simulink model "Test_Tricopter_Model"  (R2015a)
settings: Solver=ode3  SolverMode=SingleTasking  StartTime=0.0  StopTime=20  FixedStep=T_sim  RelTol=1e-3
PreLoadFcn:
  | LoadLibraries
values from neighbouring files (symbols this model uses):
  a = 10.26    [SetupComplete.m]
  A_x = 0.015    [SetupComplete.m]
  A_y = A_x    (= 0.015)    [SetupComplete.m]
  A_z = 0.16    [SetupComplete.m]
  C_d0 = 0.001193    [SetupComplete.m]
  C_x = 1.2    [SetupComplete.m]
  C_y = C_x    (= 1.2)    [SetupComplete.m]
  C_z = 2.2    [SetupComplete.m]
  CG_0 = [0,0,0.02]'    [SetupComplete.m]
  g = 9.81    [SetupComplete.m]
  h = 0.08    [SetupComplete.m]
  h_FA = 0.02    [SetupComplete.m]
  h_M = 0.064    [SetupComplete.m]
  I_BAC_0 = [ Ix,0,Ixz;0,Iy,0;Ixz,0,Iz]    [SetupComplete.m]
  I_prop = 1/4*M_eq*R^2*diag([1,1,2])    [SetupComplete.m]
  I_tube = [1/2*M_tube*R_tube_eq^2,0,  0  ;           0 ,1/3*M_tube*l_arm^2,0;             0  ,0,1/3*M_tube*l_arm^2]    [SetupComplete.m]
  Initial_Omegas = [1;1;1]*Omega_hover    [Run3Copter.m]
  J_FA = I_prop(1,1) + m_prop*h^2  + m_FA*h_FA^2 + m_M*h_M^2    [SetupComplete.m]
  J_T = J_m+1/2*M_eq*R^2    (= 2.000642e-05)    [SetupComplete.m]
  Ki = lqi(LM_4DOF_aug, Q,R)    [robust_controller.m]
  l = 0.3450    (= 0.345)    [NDI_components.m]    (also in SetupComplete.m; robust_controller.m)
  l_arm = 0.264    [SetupComplete.m]
  m = 3.51    [SetupComplete.m]
  m_0 = 2.61    [SetupComplete.m]
  m_FA = 0.02    [SetupComplete.m]
  m_M = 0.300    (= 0.3)    [SetupComplete.m]
  m_prop = 0.02    [SetupComplete.m]
  R = 0.1778    [SetupComplete.m]    (also in robust_controller.m = eye(4))
  rho = 1.15    [SetupComplete.m]
  sigma = b*c/(pi*R)    (= 0.107416159567)    [SetupComplete.m]
  T_sim = 0.01    [Run3Copter.m]
  theta_0 = 0.38397    [SetupComplete.m]
  theta_1 = -0.2967    [SetupComplete.m]
  trim_simplemodel = [0.589627915568 -2.20656039197 0 0.588313336084 0 0 0.588313330414 0 0]    [trimvalues.mat]
  V_4DOF_last = [0.0122475086001 0.00870447045314 -0.0292257707267 -0.0198753669721 -0.00290766514824 -0.0269511839788 0.0344308792695 -0.0305235710433 -0.0274078219028 -0.0329291952852 -0.0272335702183 -0.00643013158961 ... (1500 elements, 50x30)]    [NN_c_weights.mat]
  v_i0 = sqrt( 1/3*m*g/(2*rho*pi*R^2)  )    [SetupComplete.m]
  W_4DOF_last = [0.0132359246225 -0.0402459595001 -0.0221501781133 0.0046881519205 0.0457506835434 0.0464888535199 -0.0342386918322 0.0470592781761 0.0457166948243 -0.00146243512772 0.0300280468889 -0.0358113661373 ... (204 elements, 4x51)]    [NN_c_weights.mat]
undefined symbols (not defined in the file or in its folder): DOWN_0, EAST_0, Motor, NORTH_0, P_0, Prop, Q_0, R_0, sigmatest, U_0, V_0, v_i_adim, Vx_adim, Vz_adim, W_0
undefined symbols (not defined in the file): Initial_Torques, Rotation_sign, Tau_motors
libraries: simulink x61, XXCopter x32, vrlib x26, simulink_extras x6, aerolib6dofsys x3, qcatlib x3, dspinverses x3, lib_controller x2, aerolibtransform2 x2, aerolib6dof2 x1
(part 10 of 10)

== matlab function Test_Tricopter_Model/Controller/NDI+CA Controller/4DOF NDI+CA Controller - No massic update/G(X) 4DOF_WPQR1 ==
  data: gx output size=[4,4]; prev_input input size=[9,1]
function gx = gx(prev_input)
    % Calculates f_hat(x). The expression is calculated in NDI_components
    % x_dot = f(x) + g(x,u)
    %   g(x,u) ~= g(x,u0) + jac(g(x,u), u)(u0) * (u - u0)
    %   g(x,u) ~= h(x,u0) + jac(g(x,u), u)(u0) * u
    % x_dot = f_hat(x) + jac(g(x,u), u) * u
    %   f_hat(x) = f(x) + g(x,u0) - jac(g(x,u), u)(u0) *  u0
    %   g_hat(x) = jac(g(x,u), u)(u0)
    % x_dot = f_hat(x) + g_hat(x) * u
    tau1_0 = prev_input(1);
    eta1_0 = prev_input(2);
    gamma1_0 = prev_input(3);
    tau2_0 = prev_input(4);
    eta2_0 = prev_input(5);
    gamma2_0 = prev_input(6);
    tau3_0 = prev_input(7);
    eta3_0 = prev_input(8);
    gamma3_0 = prev_input(9);
    
    % This matrix was precomputed in NDI_components.m
    % TODO Precompute sines and cosines to improve performance. Some
    % repeated terms can also be precomputed
    
    % Kt = 29.6 Kq = 0.3
    gx = [...
                          -7.379*cos(eta1_0),                                7.379*tau1_0*sin(eta1_0), -7.379,  -7.379;
     0.04359*cos(eta1_0) - 1.541*sin(eta1_0), - 1.541*tau1_0*cos(eta1_0) - 0.04359*tau1_0*sin(eta1_0), -48.41,   48.32;
       43.76*cos(eta1_0) + 1.469*sin(eta1_0),     1.469*tau1_0*cos(eta1_0) - 43.76*tau1_0*sin(eta1_0), -21.88,  -21.88;
       26.0*sin(eta1_0) - 0.8729*cos(eta1_0),     26.0*tau1_0*cos(eta1_0) + 0.8729*tau1_0*sin(eta1_0),  1.997, -0.2515];
 
% Kt = 15 Kq = 0.07
%                        -4.274*cos(eta1_0),                                 4.274*tau1_0*sin(eta1_0), -4.274,  -4.274;
%  0.01017*cos(eta1_0) - 0.8926*sin(eta1_0), - 0.8926*tau1_0*cos(eta1_0) - 0.01017*tau1_0*sin(eta1_0), -28.02,    28.0;
%    25.34*cos(eta1_0) + 0.3428*sin(eta1_0),     0.3428*tau1_0*cos(eta1_0) - 25.34*tau1_0*sin(eta1_0), -12.67,  -12.67;
%    15.06*sin(eta1_0) - 0.2037*cos(eta1_0),     15.06*tau1_0*cos(eta1_0) + 0.2037*tau1_0*sin(eta1_0), 0.8549, -0.4475];

== matlab function Test_Tricopter_Model/Controller/NDI+CA Controller/4DOF NDI+CA Controller - No massic update/Rotational Kinematics ==
  data: PQR output; Eulerdot input; Euler input
function PQR = rot_kin(Eulerdot,Euler)
%solves rotational kinematic equations
Phi = Euler(1);
Theta = Euler(2);
Psi = Euler(3);
A = [1 sin(Phi)*tan(Theta) cos(Phi)*tan(Theta);
     0 cos(Phi) -sin(Phi);
     0 sin(Phi)*sec(Theta) cos(Phi)*sec(Theta)];
PQR = A'*Eulerdot;
end

== matlab function Test_Tricopter_Model/3 Copter Complete/Arms Dynamics: Forces and Moments/9 DOF Arms Dynamics: Forces and Moments/9 DOF Arms Dynamics: Forces and Moments/Arm Dynamics1/Gyroscopic Moments/Arm Inertia1 ==
  data: T_FAFb input; Arm_axis input; J_Arm output; I_tube parameter; I_prop parameter; h_FA parameter; h_M parameter; m_FA parameter; m_M parameter; m_prop parameter; h parameter
function J_Arm  = Arm_inertia(T_FAFb,Arm_axis, I_tube, I_prop, h_FA, h_M, m_FA, m_M, m_prop, h)


r_FAO=Arm_axis+T_FAFb*[0;0;-h_FA];
r_MO=Arm_axis+T_FAFb*[0;0;-h_M];
r_po=Arm_axis+T_FAFb*[0;0;-h];

I_FA = m_FA*[ r_FAO(2)^2+r_FAO(3)^2,r_FAO(1)*r_FAO(2),r_FAO(1)*r_FAO(3);...
            r_FAO(1)*r_FAO(2), r_FAO(1)^2+r_FAO(3)^2, r_FAO(2)*r_FAO(3);...
            r_FAO(1)*r_FAO(3),r_FAO(2)*r_FAO(3), r_FAO(1)^2+r_FAO(2)^2];
I_M = m_M*[ r_MO(2)^2+r_MO(3)^2,r_MO(1)*r_MO(2),r_MO(1)*r_MO(3);...
            r_MO(1)*r_MO(2), r_MO(1)^2+r_MO(3)^2, r_MO(2)*r_MO(3);...
            r_MO(1)*r_MO(3),r_MO(2)*r_MO(3), r_MO(1)^2+r_MO(2)^2];
I_steiner = m_prop*[ r_po(2)^2+r_po(3)^2,r_po(1)*r_po(2),r_po(1)*r_po(3);...
            r_po(1)*r_po(2), r_po(1)^2+r_po(3)^2, r_po(2)*r_po(3);...
            r_po(1)*r_po(3),r_po(2)*r_po(3), r_po(1)^2+r_po(2)^2];


% J_Arm = T_FAFb*I_prop*T_FAFb'+ I_tube +I_FA+I_M+I_steiner;
J_Arm = T_FAFb*I_prop*T_FAFb' +I_FA+I_M+I_steiner; % Quitamos el tubo ya que es insignificante y hay que calcularlo para cada brazo

== matlab function Test_Tricopter_Model/3 Copter Complete/Arms Dynamics: Forces and Moments/9 DOF Arms Dynamics: Forces and Moments/9 DOF Arms Dynamics: Forces and Moments/Arm Dynamics2/Gyroscopic Moments/Arm Inertia1 ==
  data: T_FAFb input; Arm_axis input; J_Arm output; I_tube parameter; I_prop parameter; h_FA parameter; h_M parameter; m_FA parameter; m_M parameter; m_prop parameter; h parameter
function J_Arm  = Arm_inertia(T_FAFb,Arm_axis, I_tube, I_prop, h_FA, h_M, m_FA, m_M, m_prop, h)


r_FAO=Arm_axis+T_FAFb*[0;0;-h_FA];
r_MO=Arm_axis+T_FAFb*[0;0;-h_M];
r_po=Arm_axis+T_FAFb*[0;0;-h];

I_FA = m_FA*[ r_FAO(2)^2+r_FAO(3)^2,r_FAO(1)*r_FAO(2),r_FAO(1)*r_FAO(3);...
            r_FAO(1)*r_FAO(2), r_FAO(1)^2+r_FAO(3)^2, r_FAO(2)*r_FAO(3);...
            r_FAO(1)*r_FAO(3),r_FAO(2)*r_FAO(3), r_FAO(1)^2+r_FAO(2)^2];
I_M = m_M*[ r_MO(2)^2+r_MO(3)^2,r_MO(1)*r_MO(2),r_MO(1)*r_MO(3);...
            r_MO(1)*r_MO(2), r_MO(1)^2+r_MO(3)^2, r_MO(2)*r_MO(3);...
            r_MO(1)*r_MO(3),r_MO(2)*r_MO(3), r_MO(1)^2+r_MO(2)^2];
I_steiner = m_prop*[ r_po(2)^2+r_po(3)^2,r_po(1)*r_po(2),r_po(1)*r_po(3);...
            r_po(1)*r_po(2), r_po(1)^2+r_po(3)^2, r_po(2)*r_po(3);...
            r_po(1)*r_po(3),r_po(2)*r_po(3), r_po(1)^2+r_po(2)^2];


% J_Arm = T_FAFb*I_prop*T_FAFb'+ I_tube +I_FA+I_M+I_steiner;
J_Arm = T_FAFb*I_prop*T_FAFb' +I_FA+I_M+I_steiner; % Quitamos el tubo ya que es insignificante y hay que calcularlo para cada brazo

== matlab function Test_Tricopter_Model/3 Copter Complete/Arms Dynamics: Forces and Moments/9 DOF Arms Dynamics: Forces and Moments/9 DOF Arms Dynamics: Forces and Moments/Arm Dynamics/Gyroscopic Moments/Arm Inertia1 ==
  data: T_FAFb input; Arm_axis input; J_Arm output; I_tube parameter; I_prop parameter; h_FA parameter; h_M parameter; m_FA parameter; m_M parameter; m_prop parameter; h parameter
function J_Arm  = Arm_inertia(T_FAFb,Arm_axis, I_tube, I_prop, h_FA, h_M, m_FA, m_M, m_prop, h)


r_FAO=Arm_axis+T_FAFb*[0;0;-h_FA];
r_MO=Arm_axis+T_FAFb*[0;0;-h_M];
r_po=Arm_axis+T_FAFb*[0;0;-h];

I_FA = m_FA*[ r_FAO(2)^2+r_FAO(3)^2,r_FAO(1)*r_FAO(2),r_FAO(1)*r_FAO(3);...
            r_FAO(1)*r_FAO(2), r_FAO(1)^2+r_FAO(3)^2, r_FAO(2)*r_FAO(3);...
            r_FAO(1)*r_FAO(3),r_FAO(2)*r_FAO(3), r_FAO(1)^2+r_FAO(2)^2];
I_M = m_M*[ r_MO(2)^2+r_MO(3)^2,r_MO(1)*r_MO(2),r_MO(1)*r_MO(3);...
            r_MO(1)*r_MO(2), r_MO(1)^2+r_MO(3)^2, r_MO(2)*r_MO(3);...
            r_MO(1)*r_MO(3),r_MO(2)*r_MO(3), r_MO(1)^2+r_MO(2)^2];
I_steiner = m_prop*[ r_po(2)^2+r_po(3)^2,r_po(1)*r_po(2),r_po(1)*r_po(3);...
            r_po(1)*r_po(2), r_po(1)^2+r_po(3)^2, r_po(2)*r_po(3);...
            r_po(1)*r_po(3),r_po(2)*r_po(3), r_po(1)^2+r_po(2)^2];


% J_Arm = T_FAFb*I_prop*T_FAFb'+ I_tube +I_FA+I_M+I_steiner;
J_Arm = T_FAFb*I_prop*T_FAFb' +I_FA+I_M+I_steiner; % Quitamos el tubo ya que es insignificante y hay que calcularlo para cada brazo
